simulink model "testBlockDiff"  (R2023b)
settings: Solver=VariableStepAuto  StartTime=0.0  StopTime=10.0  RelTol=1e-3
settings Model: Creator=neham  LastModifiedBy=neham

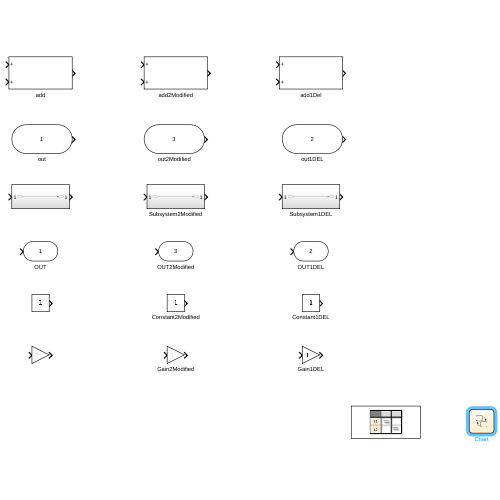
[thumbnail: Simulink's stored preview of the top-level diagram]
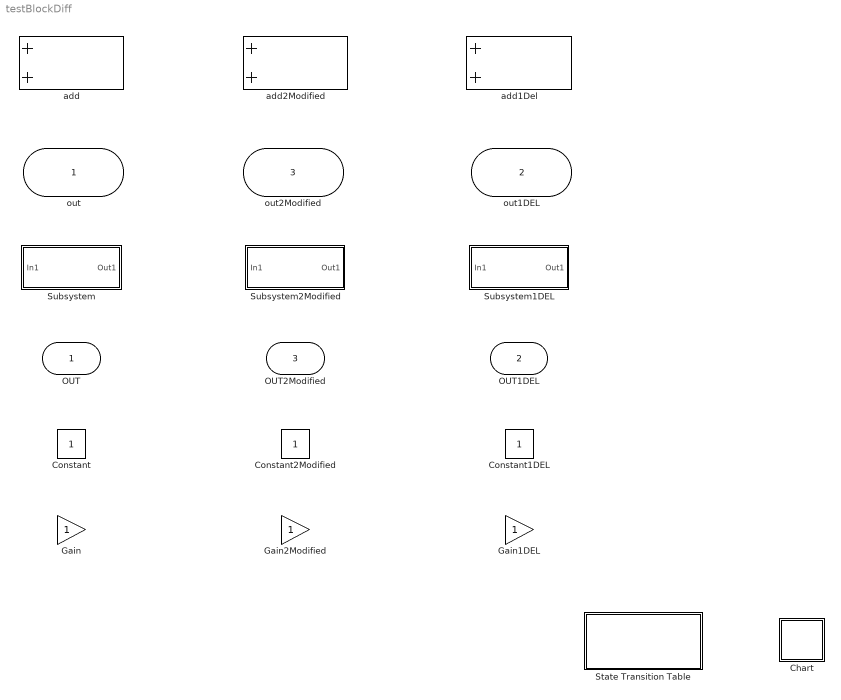
== system testBlockDiff ==
  out : Inport
  out1DEL : Inport  Port=2
  out2Modified : Inport  Port=3
  Chart : Stateflow chart  TreatAsAtomicUnit=on
  Constant : Constant
  Constant1DEL : Constant
  Constant2Modified : Constant
  Gain : Gain
  Gain1DEL : Gain
  Gain2Modified : Gain
  State Transition Table : State Transition Table  TreatAsAtomicUnit=on
  Subsystem : Subsystem
  Subsystem1DEL : Subsystem
  Subsystem2Modified : Subsystem
  add : Sum
  add1Del : Sum
  add2Modified : Sum
  OUT : Outport
  OUT1DEL : Outport  Port=2
  OUT2Modified : Outport  Port=3

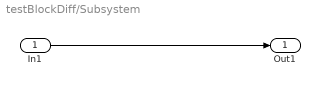
== system testBlockDiff/Subsystem ==
  In1 : Inport
  Out1 : Outport
  wires:
  In1/1 -> Out1/1

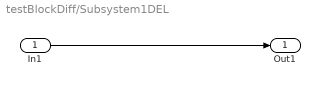
== system testBlockDiff/Subsystem1DEL ==
  In1 : Inport
  Out1 : Outport
  wires:
  In1/1 -> Out1/1

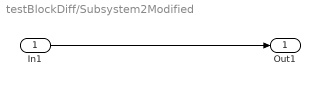
== system testBlockDiff/Subsystem2Modified ==
  In1 : Inport
  Out1 : Outport
  wires:
  In1/1 -> Out1/1

== stateflow chart testBlockDiff/Chart ==

== stateflow chart testBlockDiff/State Transition Table ==
  state state1
  state state2
  (default) -> state1
  state1 -> state2
